simulink model "VisualWarningSystem"  (R2016a)
settings: Solver=FixedStepAuto  StartTime=0.0  StopTime=10.0  RelTol=1e-3
settings Model: Creator=Josef  LastModifiedBy=Josef
settings GRTTargetCC: GeneratePreprocessorConditionals=Use local settings

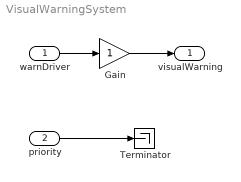
== system VisualWarningSystem ==
  warnDriver : Inport  OutDataTypeStr=boolean
      settings: AttributesFormatString=detectObstacleandWarnDriver
  priority : Inport  Port=2
      settings: AttributesFormatString=signal
  Gain : Gain  OutDataTypeStr=double
  Terminator : Terminator
  visualWarning : Outport
      settings: AttributesFormatString=provideWarning
  wires:
  warnDriver/1 -> Gain/1
  Gain/1 -> visualWarning/1
  priority/1 -> Terminator/1
